simulink model "RRRmodel_ClosedLoop"  (R2019b)
settings: Solver=ode3  StartTime=0.0  StopTime=30  FixedStep=0.01  RelTol=1e-3
undefined symbols (not defined in the file or in its folder): Kp, Kv, x_init
libraries: simulink x8
settings Model: Creator=Chris  LastModifiedBy=Chris

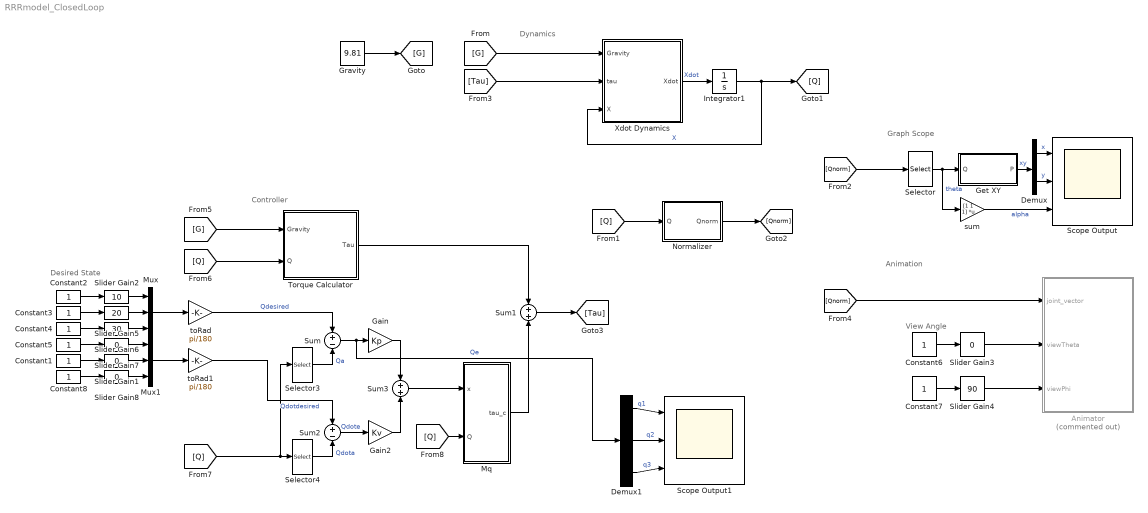
== system RRRmodel_ClosedLoop ==
  note: Controller
  note: Dynamics
  note: Animation
  note: View Angle
  note: Desired State
  note: Graph Scope
  Animator : MATLAB Function  Commented=on  TreatAsAtomicUnit=on
  Constant{1..8} (8 alike) : Constant
  Demux : Demux  Outputs=2
  Demux1 : Demux  Outputs=3
  Gain : Gain  Gain=Kp
  Gain2 : Gain  Gain=Kv
  Get XY : MATLAB Function  TreatAsAtomicUnit=on
  Gravity : Constant  Value=9.81
  Integrator1 : Integrator  InitialCondition=-x_init
  Mq : MATLAB Function  TreatAsAtomicUnit=on
  Mux : Mux  Inputs=3
  Mux1 : Mux  Inputs=3
  Normalizer : MATLAB Function  TreatAsAtomicUnit=on
  Scope Output : Scope  NumInputPorts=3
  Scope Output1 : Scope  NumInputPorts=3
  Selector : Selector  InputPortWidth=6  IndexOptions=Index vector (dialog)  Indices=[1 3 5]  OutputSizes=1
  Selector3 : Selector  InputPortWidth=6  IndexOptions=Index vector (dialog)  Indices=[1 3 5]  OutputSizes=1
  Selector4 : Selector  InputPortWidth=6  IndexOptions=Index vector (dialog)  Indices=[2 4 6]  OutputSizes=1
  Slider Gain{1,3,7..8} (4 alike) : simulink/Math Operations/Slider Gain  gain=0  low=-90  high=90
  Slider Gain2 : simulink/Math Operations/Slider Gain  gain=10  low=-90  high=90
  Slider Gain4 : simulink/Math Operations/Slider Gain  gain=90  low=-90  high=90
  Slider Gain5 : simulink/Math Operations/Slider Gain  gain=20  low=-90  high=90
  Slider Gain6 : simulink/Math Operations/Slider Gain  gain=30  low=-90  high=90
  Sum : Sum  Inputs=+|-
  Sum1 : Sum  Inputs=+|+
  Sum2 : Sum  Inputs=+|-
  Sum3 : Sum  Inputs=+|+
  Torque Calculator : MATLAB Function  TreatAsAtomicUnit=on
  Xdot Dynamics : MATLAB Function  TreatAsAtomicUnit=on
  sum : Gain  Gain=[1 1 1]  Multiplication=Matrix(K*u)
  toRad : Gain  Gain=pi/180
  toRad1 : Gain  Gain=pi/180
  wires:
  Torque Calculator/1(Tau) -> Sum1/1
  Xdot Dynamics/1(Xdot) -> Integrator1/1  "Xdot"
  Slider Gain3/1 -> Animator/2(viewTheta)
  Slider Gain4/1 -> Animator/3(viewPhi)
  Constant6/1 -> Slider Gain3/1
  Constant7/1 -> Slider Gain4/1
  Gravity/1 -> [G]
  [G] -> Xdot Dynamics/1(Gravity)
  Integrator1/1 -> Xdot Dynamics/3(X), [Q]  "X"
  [Tau] -> Xdot Dynamics/2(tau)
  [Qnorm] -> Animator/1(joint_vector)
  [G] -> Torque Calculator/1(Gravity)
  Normalizer/1(Qnorm) -> [Qnorm]
  [Q] -> Normalizer/1(Q)
  Constant3/1 -> Slider Gain5/1
  Slider Gain6/1 -> Mux/3
  Slider Gain2/1 -> Mux/1
  Constant8/1 -> Slider Gain8/1
  Constant1/1 -> Slider Gain1/1
  Slider Gain1/1 -> Mux1/2
  Constant4/1 -> Slider Gain6/1
  Constant2/1 -> Slider Gain2/1
  Slider Gain5/1 -> Mux/2
  Constant5/1 -> Slider Gain7/1
  Slider Gain7/1 -> Mux1/1
  Slider Gain8/1 -> Mux1/3
  Mux/1 -> toRad/1
  [Q] -> Selector3/1, Selector4/1
  Selector4/1 -> Sum2/2  "Qdota"
  Selector3/1 -> Sum/2  "Qa"
  Sum3/1 -> Mq/1(x)
  Sum1/1 -> [Tau]
  [Q] -> Torque Calculator/2(Q)
  toRad/1 -> Sum/1  "Qdesired"
  Sum/1 -> Demux1/1, Gain/1  "Qe"
  Sum2/1 -> Gain2/1  "Qdote"
  Gain/1 -> Sum3/1
  Gain2/1 -> Sum3/2
  Mux1/1 -> toRad1/1
  [Q] -> Mq/2(Q)
  Mq/1(tau_c) -> Sum1/2
  toRad1/1 -> Sum2/1  "Qdotdesired"
  Demux/2 -> Scope Output/2  "y"
  [Qnorm] -> Selector/1
  Get XY/1(P) -> Demux/1  "xy"
  sum/1 -> Scope Output/3  "alpha"
  Selector/1 -> sum/1, Get XY/1(Q)  "theta"
  Demux/1 -> Scope Output/1  "x"
  Demux1/1 -> Scope Output1/1  "q1"
  Demux1/2 -> Scope Output1/2  "q2"
  Demux1/3 -> Scope Output1/3  "q3"

== matlab function RRRmodel_ClosedLoop/Normalizer ==
  data: Q input; Qnorm output
function Qnorm = fcn(Q)

q = Q(1:3);
qdot = Q(4:6);
qnorm = 2.*atan(tan(q./2));

Qnorm = [qnorm;qdot];

== matlab function RRRmodel_ClosedLoop/Xdot Dynamics ==
  data: Xdot output; Gravity input; tau input; X input
function Xdot = xdot(Gravity,tau,X)

%% Unpack Variables
SFric1=0;
DFric1=200;
SFric2=0;
DFric2=150;
SFric3=0;
DFric3=100;

grav=Gravity;

q1=X(1);
q1dot=X(2);
q2=X(3);
q2dot=X(4);
q3=X(5);
q3dot=X(6);

%% Calculate Dynamics Matrices
Mq = [...
      80*cos(q2 + q3) + 420*cos(q2) + 60*cos(q3) + 12291/20, 40*cos(q2 + q3) + 210*cos(q2) + 60*cos(q3) + 2681/20, 40*cos(q2 + q3) + 30*cos(q3) + 101/10;...
       40*cos(q2 + q3) + 210*cos(q2) + 60*cos(q3) + 2681/20,                                 60*cos(q3) + 2681/20,                   30*cos(q3) + 101/10;...
                      40*cos(q2 + q3) + 30*cos(q3) + 101/10,                                  30*cos(q3) + 101/10,                                101/10;...
];


Vq = [...
      - q3dot*(40*q2dot*sin(q2 + q3) + q3dot*(40*sin(q2 + q3) + 30*sin(q3))) - q2dot*(q3dot*(40*sin(q2 + q3) + 60*sin(q3)) + q2dot*(40*sin(q2 + q3) + 210*sin(q2))) - q1dot*(q3dot*(80*sin(q2 + q3) + 60*sin(q3)) + q2dot*(80*sin(q2 + q3) + 420*sin(q2)));...
      210*q1dot^2*sin(q2) - 30*q3dot^2*sin(q3) + 40*q1dot^2*sin(q2 + q3) - 60*q1dot*q3dot*sin(q3) - 60*q2dot*q3dot*sin(q3);...
      30*q1dot^2*sin(q3) + 30*q2dot^2*sin(q3) + 40*q1dot^2*sin(q2 + q3) + 60*q1dot*q2dot*sin(q3);...
];

Gq = [...
      (5*grav*(4*cos(q1 + q2 + q3) + 21*cos(q1 + q2) + 56*cos(q1)))/2;...
      (105*grav*cos(q1 + q2))/2 + 10*grav*cos(q1 + q2 + q3);...
      10*grav*cos(q1 + q2 + q3);...
];


F1=SFric1*sign(q1dot) + DFric1*q1dot;
F2=SFric2*sign(q2dot) + DFric2*q2dot;
F3=SFric3*sign(q3dot) + DFric3*q3dot;

Fq=[F1;F2;F3];

%% Get Acceleration and Xdot
accel = Mq^(-1)*(tau - Vq - Gq - Fq);
Xdot=[q1dot;accel(1);q2dot;accel(2);q3dot;accel(3)];


end

== matlab function RRRmodel_ClosedLoop/Animator ==
  data: joint_vector input; viewTheta input; viewPhi input
function Model_Robot(joint_vector, viewTheta, viewPhi)

%% Unpack Joint Vector
theta = joint_vector;
L1 = 8;
L2 = 6;
EOA = 4;
L = [0 L1 L2 EOA];

%% Define Links/ Robot Shapes

Base  = [...
         -1  -1  -1  -1  -1   1   1  -1   1   1  -1   1   1  -1   1   1;...
          1  -1  -1   1   1   1   1   1   1  -1  -1  -1  -1  -1  -1   1;...
        -15 -15  -1  -1 -15 -15  -1  -1  -1  -1  -1  -1 -15 -15 -15 -15;...
];

Link1 = [...
          1  -1  -1   1   1   1   1   1   1  -1  -1  -1  -1  -1  -1   1;...
          1   1  -1  -1   1   1  -1  -1  -1  -1  -1  -1   1   1   1   1;...
         -1  -1  -1  -1  -1   1   1  -1   1   1  -1   1   1  -1   1   1;...
];

L1rod = [...
          1  L1  L1   1   1   1   1   1   1  L1  L1  L1  L1  L1  L1   1;...
         .5  .5 -.5 -.5  .5  .5 -.5 -.5 -.5 -.5 -.5 -.5  .5  .5  .5  .5;...
        -.5 -.5 -.5 -.5 -.5  .5  .5 -.5  .5  .5 -.5  .5  .5 -.5  .5  .5;...
];

Link2 = [...
          1  -1  -1   1   1   1   1   1   1  -1  -1  -1  -1  -1  -1   1;...
          1   1  -1  -1   1   1  -1  -1  -1  -1  -1  -1   1   1   1   1;...
         -1  -1  -1  -1  -1   1   1  -1   1   1  -1   1   1  -1   1   1;...
];

L2rod = [...
          1  L2  L2   1   1   1   1   1   1  L2  L2  L2  L2  L2  L2   1;...
         .5  .5 -.5 -.5  .5  .5 -.5 -.5 -.5 -.5 -.5 -.5  .5  .5  .5  .5;...
        -.5 -.5 -.5 -.5 -.5  .5  .5 -.5  .5  .5 -.5  .5  .5 -.5  .5  .5;...
];

Link3 = [...
          1  -1  -1   1   1   1   1   1   1  -1  -1  -1  -1  -1  -1   1;...
          1   1  -1  -1   1   1  -1  -1  -1  -1  -1  -1   1   1   1   1;...
         -1  -1  -1  -1  -1   1   1  -1   1   1  -1   1   1  -1   1   1;...
];

L3rod = [...
          1  EOA EOA  1   1   1   1   1   1  EOA EOA EOA EOA EOA EOA  1;...
         .5  .5 -.5 -.5  .5  .5 -.5 -.5 -.5 -.5 -.5 -.5  .5  .5  .5  .5;...
        -.5 -.5 -.5 -.5 -.5  .5  .5 -.5  .5  .5 -.5  .5  .5 -.5  .5  .5;...
];


%% Transform Link 1
BaseLink1= TRANSRRR(Link1 ,theta(1), L(1));
Link1rod = TRANSRRR(L1rod ,theta(1), L(1));

%% Transform Link 2
Link12   = TRANSRRR(Link2 ,theta(2), L(2));
BaseLink2= TRANSRRR(Link12,theta(1), L(1));

L2rod    = TRANSRRR(L2rod ,theta(2), L(2));
Link2rod = TRANSRRR(L2rod ,theta(1), L(1));

%% Transform Link 3
Link23   = TRANSRRR(Link3 ,theta(3), L(3));
Link13   = TRANSRRR(Link23,theta(2), L(2));
BaseLink3= TRANSRRR(Link13,theta(1), L(1));

L3rod    = TRANSRRR(L3rod ,theta(3), L(3));
L3rod    = TRANSRRR(L3rod ,theta(2), L(2));
Link3rod = TRANSRRR(L3rod ,theta(1), L(1));


%% Plotting
plot3(Base(1,:),Base(2,:),Base(3,:),'k-')
axis([-20 20 -20 20 -20 20]);
grid on
hold on
plot3(BaseLink1(1,:),BaseLink1(2,:),BaseLink1(3,:),'b-', 'LineWidth', 2)
plot3(Link1rod(1,:), Link1rod(2,:), Link1rod(3,:), 'b-', 'LineWidth', 2)
plot3(BaseLink2(1,:),BaseLink2(2,:),BaseLink2(3,:),'g-', 'LineWidth', 2)
plot3(Link2rod(1,:), Link2rod(2,:), Link2rod(3,:), 'g-', 'LineWidth', 2)
plot3(BaseLink3(1,:),BaseLink3(2,:),BaseLink3(3,:),'k-', 'LineWidth', 2)
plot3(Link3rod(1,:), Link3rod(2,:), Link3rod(3,:), 'k-', 'LineWidth', 2)

xlabel('X');
ylabel('Y');
zlabel('Z');
view(viewTheta,viewPhi);
set(gcf,'color','w');
hold off

end

== matlab function RRRmodel_ClosedLoop/Torque Calculator ==
  data: Tau output; Gravity input; Q input
function Tau = tau_calc(Gravity,Q)

SFric1=0;
DFric1=200;
SFric2=0;
DFric2=150;
SFric3=0;
DFric3=100;

grav=Gravity;

q1 = Q(1);
q2 = Q(3);
q3 = Q(5);
q1dot = Q(2);
q2dot = Q(4);
q3dot = Q(6);

Vq = [...
      - q3dot*(40*q2dot*sin(q2 + q3) + q3dot*(40*sin(q2 + q3) + 30*sin(q3))) - q2dot*(q3dot*(40*sin(q2 + q3) + 60*sin(q3)) + q2dot*(40*sin(q2 + q3) + 210*sin(q2))) - q1dot*(q3dot*(80*sin(q2 + q3) + 60*sin(q3)) + q2dot*(80*sin(q2 + q3) + 420*sin(q2)));...
      210*q1dot^2*sin(q2) - 30*q3dot^2*sin(q3) + 40*q1dot^2*sin(q2 + q3) - 60*q1dot*q3dot*sin(q3) - 60*q2dot*q3dot*sin(q3);...
      30*q1dot^2*sin(q3) + 30*q2dot^2*sin(q3) + 40*q1dot^2*sin(q2 + q3) + 60*q1dot*q2dot*sin(q3);...
];

Gq = [...
      (5*grav*(4*cos(q1 + q2 + q3) + 21*cos(q1 + q2) + 56*cos(q1)))/2;...
      (105*grav*cos(q1 + q2))/2 + 10*grav*cos(q1 + q2 + q3);...
      10*grav*cos(q1 + q2 + q3);...
];


F1=SFric1*sign(q1dot) + DFric1*q1dot;
F2=SFric2*sign(q2dot) + DFric2*q2dot;
F3=SFric3*sign(q3dot) + DFric3*q3dot;
Fq=[F1;F2;F3];

Tau = Vq + Gq + Fq;

end

== matlab function RRRmodel_ClosedLoop/Mq ==
  data: x input; Q input; tau_c output
function tau_c = fcn(x,Q)

q1=Q(1);
q2=Q(2);
q3=Q(3);

Mq = [...
      80*cos(q2 + q3) + 420*cos(q2) + 60*cos(q3) + 12291/20, 40*cos(q2 + q3) + 210*cos(q2) + 60*cos(q3) + 2681/20, 40*cos(q2 + q3) + 30*cos(q3) + 101/10;...
       40*cos(q2 + q3) + 210*cos(q2) + 60*cos(q3) + 2681/20,                                 60*cos(q3) + 2681/20,                   30*cos(q3) + 101/10;...
                      40*cos(q2 + q3) + 30*cos(q3) + 101/10,                                  30*cos(q3) + 101/10,                                101/10;...
];

tau_c = Mq*x;

== matlab function RRRmodel_ClosedLoop/Get XY ==
  data: Q input; P output
function P   = TRANSRRR04(Q)

q1 = Q(1);
q2 = Q(2);
q3 = Q(3);

T01 = [...
       cos(q1)  -sin(q1)  0  0 ;...
       sin(q1)   cos(q1)  0  0 ;...
         0         0      1  0 ;...
         0         0      0  1 ;...
];


T12 = [...
       cos(q2)  -sin(q2)  0  4 ;...
       sin(q2)   cos(q2)  0  0 ;...
         0         0      1  0 ;...
         0         0      0  1 ;...
];

T23 = [...
       cos(q3)  -sin(q3)  0  3 ;...
       sin(q3)   cos(q3)  0  0 ;...
         0         0      1  0 ;...
         0         0      0  1 ;...
];

T34 = [...
         1         0      0  2 ;...
         0         1      0  0 ;...
         0         0      1  0 ;...
         0         0      0  1 ;...
];

T04 = T01*T12*T23*T34;
Pt = T04*[0;0;0;1];
P = [Pt(1); Pt(2)];
end
